simulink model "busSelectorSwitch"  (R2023b)
settings: Solver=VariableStepAuto  StartTime=0.0  StopTime=10.0  RelTol=1e-3
settings Model: Creator=NITRO  LastModifiedBy=NITRO

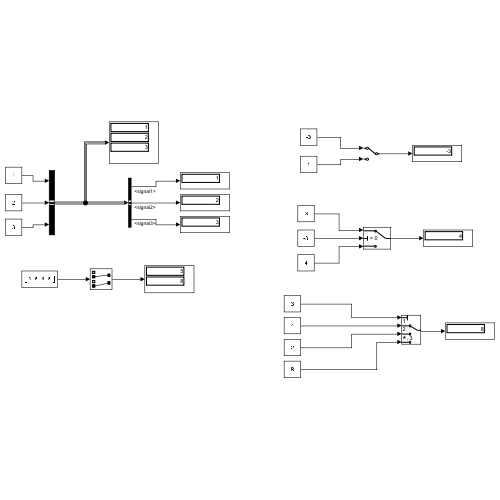
[thumbnail: Simulink's stored preview of the top-level diagram]
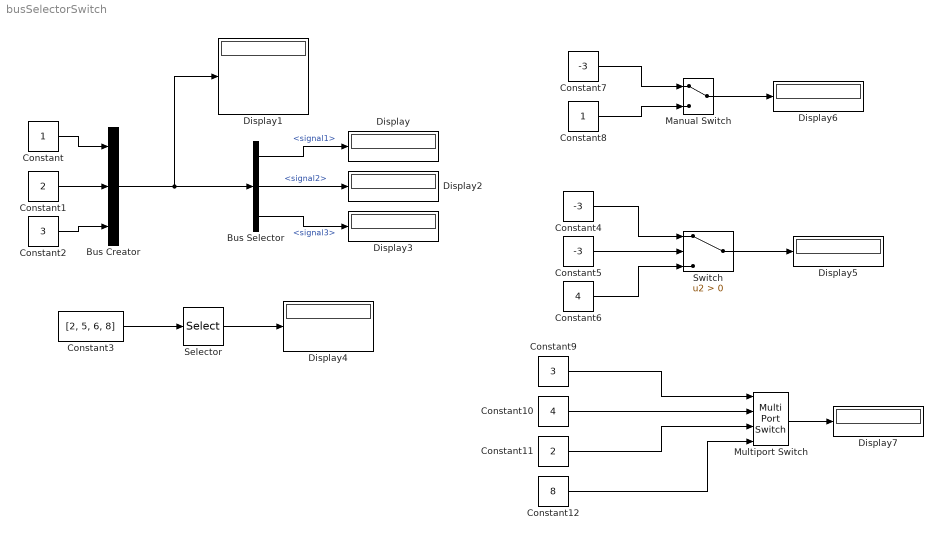
== system busSelectorSwitch ==
  Bus Creator : BusCreator  Inputs=3
  Bus Selector : BusSelector  OutputSignals=signal1,signal2,signal3
  Constant : Constant
  Constant1 : Constant  Value=2
  Constant10 : Constant  Value=4
  Constant11 : Constant  Value=2
  Constant12 : Constant  Value=8
  Constant2 : Constant  Value=3
  Constant3 : Constant  Value=[2, 5, 6, 8]
  Constant4 : Constant  Value=-3
  Constant5 : Constant  Value=-3
  Constant6 : Constant  Value=4
  Constant7 : Constant  Value=-3
  Constant8 : Constant
  Constant9 : Constant  Value=3
  Display{,1..7} (8 alike) : Display
  Manual Switch : ManualSwitch
  Multiport Switch : MultiPortSwitch  SaturateOnIntegerOverflow=off  InputSameDT=off
  Selector : Selector  InputPortWidth=4  IndexOptions=Index vector (dialog)  Indices=[2 4]  OutputSizes=1
  Switch : Switch  Criteria=u2 > Threshold  SaturateOnIntegerOverflow=off  InputSameDT=off
  wires:
  Constant1/1 -> Bus Creator/2
  Constant2/1 -> Bus Creator/3
  Constant/1 -> Bus Creator/1
  Bus Creator/1 -> Display1/1, Bus Selector/1
  Bus Selector/1 -> Display/1  "<signal1>"
  Bus Selector/2 -> Display2/1  "<signal2>"
  Bus Selector/3 -> Display3/1  "<signal3>"
  Selector/1 -> Display4/1
  Constant3/1 -> Selector/1
  Constant6/1 -> Switch/3
  Constant4/1 -> Switch/1
  Constant5/1 -> Switch/2
  Switch/1 -> Display5/1
  Manual Switch/1 -> Display6/1
  Constant7/1 -> Manual Switch/1
  Constant8/1 -> Manual Switch/2
  Multiport Switch/1 -> Display7/1
  Constant9/1 -> Multiport Switch/1
  Constant10/1 -> Multiport Switch/2
  Constant11/1 -> Multiport Switch/3
  Constant12/1 -> Multiport Switch/4
